simulink model "b_2x_8a_r309b"  (Simulink 6.2)
settings: Solver=ode45  StartTime=0.0  StopTime=1030.0  RelTol=1e-3
undefined symbols (not defined in the file): ant_bits, BEE2_usr, blockCountBits, blockRowBits, cmult_4bit_em
libraries: xbsIndex_r3 x3291, xps_library x101, casper_library x95
(part 2 of 22)

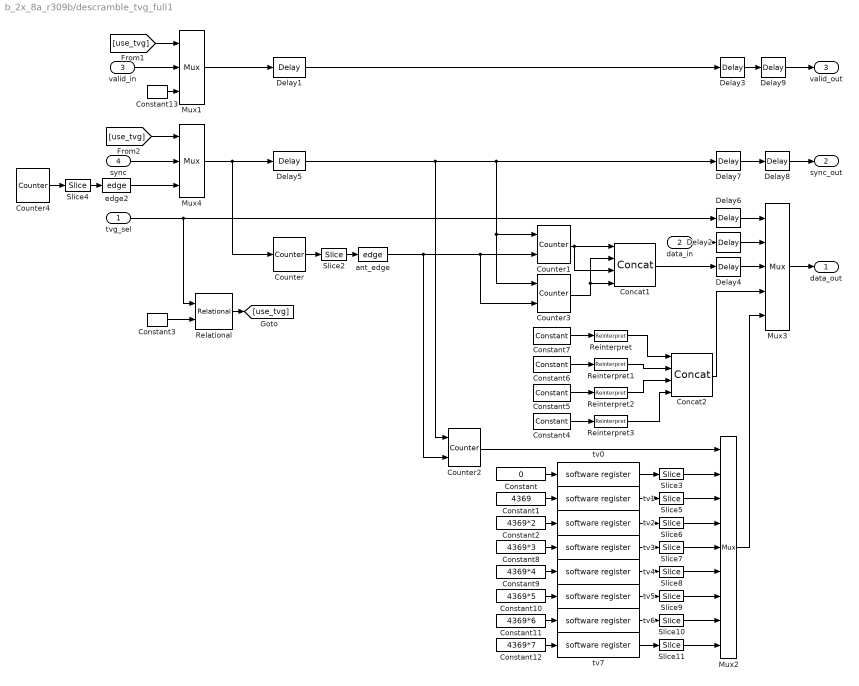
== system b_2x_8a_r309b/descramble_tvg_full1 ==
  tvg_sel : Inport  Port=1  LatchInput=off
  data_in : Inport  Port=2  LatchInput=off
  valid_in : Inport  Port=3  LatchInput=off
  sync : Inport  Port=4  LatchInput=off
  Concat1 : xbsIndex_r3/Concat  num_inputs=4  explicit_period=off  period=1  dbl_ovrd=off
  Concat2 : xbsIndex_r3/Concat  num_inputs=4  explicit_period=off  period=1  dbl_ovrd=off
  Constant : Constant  Value=0
  Constant1 : Constant  Value=4369
  Constant10 : Constant  Value=4369*5
  Constant11 : Constant  Value=4369*6
  Constant12 : Constant  Value=4369*7
  Constant13 : xbsIndex_r3/Constant  const=1  equ=P=C  arith_type=Boolean  n_bits=1  bin_pt=0  opselect=C  inp2=PCIN>>17  opr=+  inp1=P  carry=CIN  iostate=0  explicit_period=on  period=1  dbl_ovrd=off
  Constant2 : Constant  Value=4369*2
  Constant3 : xbsIndex_r3/Constant  const=0  equ=P=C  arith_type=Unsigned  n_bits=2  bin_pt=0  opselect=C  inp2=PCIN>>17  opr=+  inp1=P  carry=CIN  iostate=0  explicit_period=on  period=1  dbl_ovrd=off
  Constant4 : xbsIndex_r3/Constant  const=-0.25  equ=P=C  arith_type="Signed  (2's comp)"  n_bits=4  bin_pt=3  opselect=C  inp2=PCIN>>17  opr=+  inp1=P  carry=CIN  iostate=0  explicit_period=on  period=1  dbl_ovrd=off
  Constant5 : xbsIndex_r3/Constant  const=0.5  equ=P=C  arith_type="Signed  (2's comp)"  n_bits=4  bin_pt=3  opselect=C  inp2=PCIN>>17  opr=+  inp1=P  carry=CIN  iostate=0  explicit_period=on  period=1  dbl_ovrd=off
  Constant6 : xbsIndex_r3/Constant  const=-6/8  equ=P=C  arith_type="Signed  (2's comp)"  n_bits=4  bin_pt=3  opselect=C  inp2=PCIN>>17  opr=+  inp1=P  carry=CIN  iostate=0  explicit_period=on  period=1  dbl_ovrd=off
  Constant7 : xbsIndex_r3/Constant  const=0.1  equ=P=C  arith_type="Signed  (2's comp)"  n_bits=4  bin_pt=3  opselect=C  inp2=PCIN>>17  opr=+  inp1=P  carry=CIN  iostate=0  explicit_period=on  period=1  dbl_ovrd=off
  Constant8 : Constant  Value=4369*3
  Constant9 : Constant  Value=4369*4
  Counter : xbsIndex_r3/Counter  cnt_type=Free Running  n_bits=x_int_bits + 1  bin_pt=0  arith_type=Unsigned  start_count=0  cnt_to=Inf  cnt_by_val=1  operation=Up  explicit_period=off  period=1  load_pin=off  rst=on  en=off  dbl_ovrd=off  show_param=off  use_rpm=on  gen_core=off
      settings: xl_area=[0, 0, 0, 0, 0, 0, 0]
  Counter1 : xbsIndex_r3/Counter  cnt_type=Free Running  n_bits=4  bin_pt=0  arith_type=Unsigned  start_count=0  cnt_to=7  cnt_by_val=1  operation=Up  explicit_period=off  period=1  load_pin=off  rst=on  en=on  dbl_ovrd=off  show_param=off  use_rpm=on  gen_core=off
      settings: xl_area=[0, 0, 0, 0, 0, 0, 0]
  Counter2 : xbsIndex_r3/Counter  cnt_type=Free Running  n_bits=3  bin_pt=0  arith_type=Unsigned  start_count=0  cnt_to=7  cnt_by_val=1  operation=Up  explicit_period=off  period=1  load_pin=off  rst=on  en=on  dbl_ovrd=off  show_param=off  use_rpm=on  gen_core=off
      settings: xl_area=[0, 0, 0, 0, 0, 0, 0]
  Counter3 : xbsIndex_r3/Counter  cnt_type=Free Running  n_bits=4  bin_pt=0  arith_type=Unsigned  start_count=15  cnt_to=0  cnt_by_val=1  operation=Down  explicit_period=off  period=1  load_pin=off  rst=on  en=on  dbl_ovrd=off  show_param=off  use_rpm=on  gen_core=off
      settings: xl_area=[0, 0, 0, 0, 0, 0, 0]
  Counter4 : xbsIndex_r3/Counter  cnt_type=Free Running  n_bits=sync_period+1  bin_pt=0  arith_type=Unsigned  start_count=2^sync_period - 2  cnt_to=Inf  cnt_by_val=1  operation=Up  explicit_period=off  period=1  load_pin=off  rst=off  en=off  dbl_ovrd=off  show_param=off  use_rpm=on  gen_core=off
      settings: xl_area=[0, 0, 0, 0, 0, 0, 0]
  Delay{1,3..9} (8 alike) : xbsIndex_r3/Delay  latency=1  reg_retiming=off  explicit_period=off  period=1  en=off  accept_only_valid=off  init_zero=on  dbl_ovrd=off  show_param=off
      settings: xl_area=[0, 0, 0, 0, 0, 0, 0]
  Delay2 : xbsIndex_r3/Delay  latency=2  reg_retiming=off  explicit_period=off  period=1  en=off  accept_only_valid=off  init_zero=on  dbl_ovrd=off  show_param=off
      settings: xl_area=[0, 0, 0, 0, 0, 0, 0]
  Mux1 : xbsIndex_r3/Mux  inputs=2  precision=Full  arith_type="Signed  (2's comp)"  n_bits=8  bin_pt=2  quantization=Truncate  overflow=Wrap  latency=0  explicit_period=on  period=1  en=off  dbl_ovrd=off  show_param=off  mux_type=off  use_rpm=off  gen_core=off
      settings: xl_area=[0, 0, 0, 0, 0, 0, 0]
  Mux2 : xbsIndex_r3/Mux  inputs=8  precision=Full  arith_type="Signed  (2's comp)"  n_bits=8  bin_pt=2  quantization=Truncate  overflow=Wrap  latency=1  explicit_period=off  period=1  en=off  dbl_ovrd=off  show_param=off  mux_type=off  use_rpm=off  gen_core=off
      settings: xl_area=[0, 0, 0, 0, 0, 0, 0]
  Mux3 : xbsIndex_r3/Mux  inputs=4  precision=Full  arith_type="Signed  (2's comp)"  n_bits=8  bin_pt=2  quantization=Truncate  overflow=Wrap  latency=1  explicit_period=off  period=1  en=off  dbl_ovrd=off  show_param=off  mux_type=off  use_rpm=off  gen_core=off
      settings: xl_area=[0, 0, 0, 0, 0, 0, 0]
  Mux4 : xbsIndex_r3/Mux  inputs=2  precision=Full  arith_type="Signed  (2's comp)"  n_bits=8  bin_pt=2  quantization=Truncate  overflow=Wrap  latency=0  explicit_period=on  period=1  en=off  dbl_ovrd=off  show_param=off  mux_type=off  use_rpm=off  gen_core=off
      settings: xl_area=[0, 0, 0, 0, 0, 0, 0]
  Reinterpret{,1..3} (4 alike) : xbsIndex_r3/Reinterpret  force_arith_type=on  arith_type=Unsigned  force_bin_pt=on  bin_pt=0  force_valid=on
  Relational : xbsIndex_r3/Relational  mode=a!=b  latency=1  explicit_period=off  period=1  en=off  dbl_ovrd=off  show_param=off
      settings: xl_area=[0, 0, 0, 0, 0, 0, 0]
  Slice{3,5..11} (8 alike) : xbsIndex_r3/Slice  mode=Lower Bit Location + Width  nbits=16  bit1=0  base1=MSB of Input  bit0=0  base0=LSB of Input  boolean_output=off  explicit_period=off  period=1  dbl_ovrd=off
  Slice2 : xbsIndex_r3/Slice  mode=Lower Bit Location + Width  nbits=1  bit1=0  base1=MSB of Input  bit0=x_int_bits  base0=LSB of Input  boolean_output=on  explicit_period=off  period=1  dbl_ovrd=off
  Slice4 : xbsIndex_r3/Slice  mode=Lower Bit Location + Width  nbits=1  bit1=0  base1=MSB of Input  bit0=sync_period  base0=LSB of Input  boolean_output=on  explicit_period=off  period=1  dbl_ovrd=off
  ant_edge : casper_library/Misc/edge
  edge2 : casper_library/Misc/edge
  tv0 : xps_library/software register  Tag=xps:sw_reg  io_dir=From Processor  arith_type=Unsigned  bitwidth=32  bin_pt=0  sample_period=1  gw_name=b_2x_8a_r309b_descramble_tvg_full1_tv0_user_data_out
  tv1 : xps_library/software register  Tag=xps:sw_reg  io_dir=From Processor  arith_type=Unsigned  bitwidth=32  bin_pt=0  sample_period=1  gw_name=b_2x_8a_r309b_descramble_tvg_full1_tv1_user_data_out
  tv2 : xps_library/software register  Tag=xps:sw_reg  io_dir=From Processor  arith_type=Unsigned  bitwidth=32  bin_pt=0  sample_period=1  gw_name=b_2x_8a_r309b_descramble_tvg_full1_tv2_user_data_out
  tv3 : xps_library/software register  Tag=xps:sw_reg  io_dir=From Processor  arith_type=Unsigned  bitwidth=32  bin_pt=0  sample_period=1  gw_name=b_2x_8a_r309b_descramble_tvg_full1_tv3_user_data_out
  tv4 : xps_library/software register  Tag=xps:sw_reg  io_dir=From Processor  arith_type=Unsigned  bitwidth=32  bin_pt=0  sample_period=1  gw_name=b_2x_8a_r309b_descramble_tvg_full1_tv4_user_data_out
  tv5 : xps_library/software register  Tag=xps:sw_reg  io_dir=From Processor  arith_type=Unsigned  bitwidth=32  bin_pt=0  sample_period=1  gw_name=b_2x_8a_r309b_descramble_tvg_full1_tv5_user_data_out
  tv6 : xps_library/software register  Tag=xps:sw_reg  io_dir=From Processor  arith_type=Unsigned  bitwidth=32  bin_pt=0  sample_period=1  gw_name=b_2x_8a_r309b_descramble_tvg_full1_tv6_user_data_out
  tv7 : xps_library/software register  Tag=xps:sw_reg  io_dir=From Processor  arith_type=Unsigned  bitwidth=32  bin_pt=0  sample_period=1  gw_name=b_2x_8a_r309b_descramble_tvg_full1_tv7_user_data_out
  data_out : Outport
  sync_out : Outport  Port=2
  valid_out : Outport  Port=3
  wires:
  Counter1/1 -> Concat1/1, Concat1/3
  ant_edge/1 -> Counter2/2, Counter1/2, Counter3/2
  Counter/1 -> Slice2/1
  Slice2/1 -> ant_edge/1
  Concat1/1 -> Delay4/1
  Delay8/1 -> sync_out/1
  data_in/1 -> Delay2/1
  Delay2/1 -> Mux3/2
  Mux3/1 -> data_out/1
  Delay3/1 -> Delay9/1
  tvg_sel/1 -> Delay6/1, Relational/1
  Delay6/1 -> Mux3/1
  Constant3/1 -> Relational/2
  Concat2/1 -> Mux3/4
  Counter3/1 -> Concat1/2, Concat1/4
  Delay7/1 -> Delay8/1
  Delay5/1 -> Delay7/1, Counter1/1, Counter3/1, Counter2/1
  Delay4/1 -> Mux3/3
  Relational/1 -> [use_tvg]
  [use_tvg] -> Mux4/1
  Slice4/1 -> edge2/1
  Counter4/1 -> Slice4/1
  sync/1 -> Mux4/2
  Mux4/1 -> Delay5/1, Counter/1
  tv0/1 -> Slice3/1
  Constant/1 -> tv0/1
  Mux2/1 -> Mux3/5
  Slice3/1 -> Mux2/2
  Counter2/1 -> Mux2/1
  tv1/1 -> Slice5/1
  tv2/1 -> Slice6/1
  tv3/1 -> Slice7/1
  tv4/1 -> Slice8/1
  tv5/1 -> Slice9/1
  tv6/1 -> Slice10/1
  tv7/1 -> Slice11/1
  Slice5/1 -> Mux2/3
  Slice6/1 -> Mux2/4
  Slice7/1 -> Mux2/5
  Slice8/1 -> Mux2/6
  Slice9/1 -> Mux2/7
  Slice10/1 -> Mux2/8
  Slice11/1 -> Mux2/9
  edge2/1 -> Mux4/3
  Constant7/1 -> Reinterpret/1
  Constant6/1 -> Reinterpret1/1
  Constant5/1 -> Reinterpret2/1
  Constant4/1 -> Reinterpret3/1
  Reinterpret/1 -> Concat2/1
  Reinterpret1/1 -> Concat2/2
  Reinterpret2/1 -> Concat2/3
  Reinterpret3/1 -> Concat2/4
  Constant1/1 -> tv1/1
  Constant2/1 -> tv2/1
  Constant12/1 -> tv7/1
  Constant11/1 -> tv6/1
  Constant10/1 -> tv5/1
  Constant9/1 -> tv4/1
  Constant8/1 -> tv3/1
  Delay9/1 -> valid_out/1
  valid_in/1 -> Mux1/2
  Mux1/1 -> Delay1/1
  [use_tvg] -> Mux1/1
  Constant13/1 -> Mux1/3
  Delay1/1 -> Delay3/1

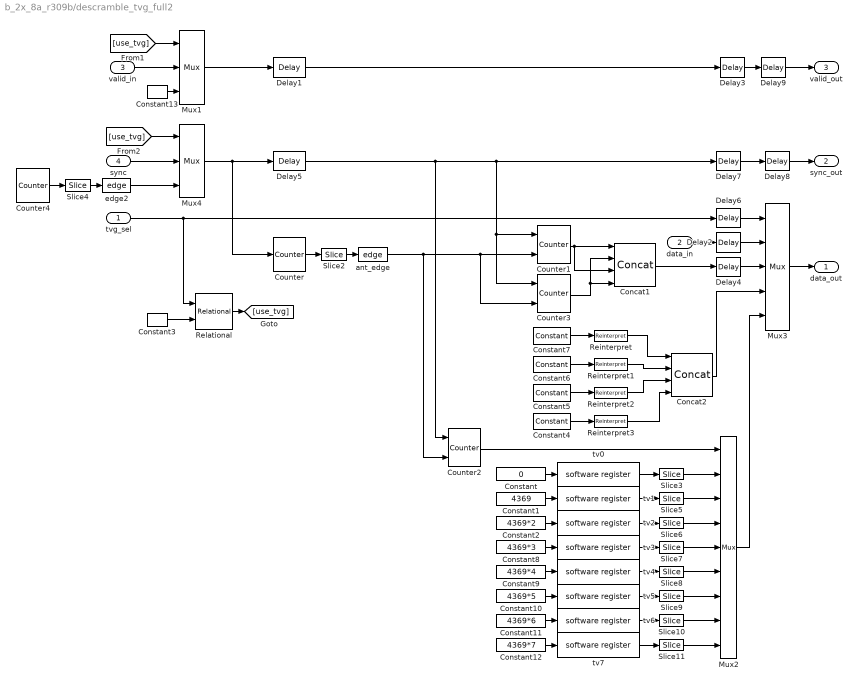
== system b_2x_8a_r309b/descramble_tvg_full2 ==
  tvg_sel : Inport  Port=1  LatchInput=off
  data_in : Inport  Port=2  LatchInput=off
  valid_in : Inport  Port=3  LatchInput=off
  sync : Inport  Port=4  LatchInput=off
  Concat1 : xbsIndex_r3/Concat  num_inputs=4  explicit_period=off  period=1  dbl_ovrd=off
  Concat2 : xbsIndex_r3/Concat  num_inputs=4  explicit_period=off  period=1  dbl_ovrd=off
  Constant : Constant  Value=0
  Constant1 : Constant  Value=4369
  Constant10 : Constant  Value=4369*5
  Constant11 : Constant  Value=4369*6
  Constant12 : Constant  Value=4369*7
  Constant13 : xbsIndex_r3/Constant  const=1  equ=P=C  arith_type=Boolean  n_bits=1  bin_pt=0  opselect=C  inp2=PCIN>>17  opr=+  inp1=P  carry=CIN  iostate=0  explicit_period=on  period=1  dbl_ovrd=off
  Constant2 : Constant  Value=4369*2
  Constant3 : xbsIndex_r3/Constant  const=0  equ=P=C  arith_type=Unsigned  n_bits=2  bin_pt=0  opselect=C  inp2=PCIN>>17  opr=+  inp1=P  carry=CIN  iostate=0  explicit_period=on  period=1  dbl_ovrd=off
  Constant4 : xbsIndex_r3/Constant  const=-0.25  equ=P=C  arith_type="Signed  (2's comp)"  n_bits=4  bin_pt=3  opselect=C  inp2=PCIN>>17  opr=+  inp1=P  carry=CIN  iostate=0  explicit_period=on  period=1  dbl_ovrd=off
  Constant5 : xbsIndex_r3/Constant  const=0.5  equ=P=C  arith_type="Signed  (2's comp)"  n_bits=4  bin_pt=3  opselect=C  inp2=PCIN>>17  opr=+  inp1=P  carry=CIN  iostate=0  explicit_period=on  period=1  dbl_ovrd=off
  Constant6 : xbsIndex_r3/Constant  const=-6/8  equ=P=C  arith_type="Signed  (2's comp)"  n_bits=4  bin_pt=3  opselect=C  inp2=PCIN>>17  opr=+  inp1=P  carry=CIN  iostate=0  explicit_period=on  period=1  dbl_ovrd=off
  Constant7 : xbsIndex_r3/Constant  const=0.1  equ=P=C  arith_type="Signed  (2's comp)"  n_bits=4  bin_pt=3  opselect=C  inp2=PCIN>>17  opr=+  inp1=P  carry=CIN  iostate=0  explicit_period=on  period=1  dbl_ovrd=off
  Constant8 : Constant  Value=4369*3
  Constant9 : Constant  Value=4369*4
  Counter : xbsIndex_r3/Counter  cnt_type=Free Running  n_bits=x_int_bits + 1  bin_pt=0  arith_type=Unsigned  start_count=0  cnt_to=Inf  cnt_by_val=1  operation=Up  explicit_period=off  period=1  load_pin=off  rst=on  en=off  dbl_ovrd=off  show_param=off  use_rpm=on  gen_core=off
      settings: xl_area=[0, 0, 0, 0, 0, 0, 0]
  Counter1 : xbsIndex_r3/Counter  cnt_type=Free Running  n_bits=4  bin_pt=0  arith_type=Unsigned  start_count=0  cnt_to=7  cnt_by_val=1  operation=Up  explicit_period=off  period=1  load_pin=off  rst=on  en=on  dbl_ovrd=off  show_param=off  use_rpm=on  gen_core=off
      settings: xl_area=[0, 0, 0, 0, 0, 0, 0]
  Counter2 : xbsIndex_r3/Counter  cnt_type=Free Running  n_bits=3  bin_pt=0  arith_type=Unsigned  start_count=0  cnt_to=7  cnt_by_val=1  operation=Up  explicit_period=off  period=1  load_pin=off  rst=on  en=on  dbl_ovrd=off  show_param=off  use_rpm=on  gen_core=off
      settings: xl_area=[0, 0, 0, 0, 0, 0, 0]
  Counter3 : xbsIndex_r3/Counter  cnt_type=Free Running  n_bits=4  bin_pt=0  arith_type=Unsigned  start_count=15  cnt_to=0  cnt_by_val=1  operation=Down  explicit_period=off  period=1  load_pin=off  rst=on  en=on  dbl_ovrd=off  show_param=off  use_rpm=on  gen_core=off
      settings: xl_area=[0, 0, 0, 0, 0, 0, 0]
  Counter4 : xbsIndex_r3/Counter  cnt_type=Free Running  n_bits=sync_period+1  bin_pt=0  arith_type=Unsigned  start_count=2^sync_period - 2  cnt_to=Inf  cnt_by_val=1  operation=Up  explicit_period=off  period=1  load_pin=off  rst=off  en=off  dbl_ovrd=off  show_param=off  use_rpm=on  gen_core=off
      settings: xl_area=[0, 0, 0, 0, 0, 0, 0]
  Delay{1,3..9} (8 alike) : xbsIndex_r3/Delay  latency=1  reg_retiming=off  explicit_period=off  period=1  en=off  accept_only_valid=off  init_zero=on  dbl_ovrd=off  show_param=off
      settings: xl_area=[0, 0, 0, 0, 0, 0, 0]
  Delay2 : xbsIndex_r3/Delay  latency=2  reg_retiming=off  explicit_period=off  period=1  en=off  accept_only_valid=off  init_zero=on  dbl_ovrd=off  show_param=off
      settings: xl_area=[0, 0, 0, 0, 0, 0, 0]
  Mux1 : xbsIndex_r3/Mux  inputs=2  precision=Full  arith_type="Signed  (2's comp)"  n_bits=8  bin_pt=2  quantization=Truncate  overflow=Wrap  latency=0  explicit_period=on  period=1  en=off  dbl_ovrd=off  show_param=off  mux_type=off  use_rpm=off  gen_core=off
      settings: xl_area=[0, 0, 0, 0, 0, 0, 0]
  Mux2 : xbsIndex_r3/Mux  inputs=8  precision=Full  arith_type="Signed  (2's comp)"  n_bits=8  bin_pt=2  quantization=Truncate  overflow=Wrap  latency=1  explicit_period=off  period=1  en=off  dbl_ovrd=off  show_param=off  mux_type=off  use_rpm=off  gen_core=off
      settings: xl_area=[0, 0, 0, 0, 0, 0, 0]
  Mux3 : xbsIndex_r3/Mux  inputs=4  precision=Full  arith_type="Signed  (2's comp)"  n_bits=8  bin_pt=2  quantization=Truncate  overflow=Wrap  latency=1  explicit_period=off  period=1  en=off  dbl_ovrd=off  show_param=off  mux_type=off  use_rpm=off  gen_core=off
      settings: xl_area=[0, 0, 0, 0, 0, 0, 0]
  Mux4 : xbsIndex_r3/Mux  inputs=2  precision=Full  arith_type="Signed  (2's comp)"  n_bits=8  bin_pt=2  quantization=Truncate  overflow=Wrap  latency=0  explicit_period=on  period=1  en=off  dbl_ovrd=off  show_param=off  mux_type=off  use_rpm=off  gen_core=off
      settings: xl_area=[0, 0, 0, 0, 0, 0, 0]
  Reinterpret{,1..3} (4 alike) : xbsIndex_r3/Reinterpret  force_arith_type=on  arith_type=Unsigned  force_bin_pt=on  bin_pt=0  force_valid=on
  Relational : xbsIndex_r3/Relational  mode=a!=b  latency=1  explicit_period=off  period=1  en=off  dbl_ovrd=off  show_param=off
      settings: xl_area=[0, 0, 0, 0, 0, 0, 0]
  Slice{3,5..11} (8 alike) : xbsIndex_r3/Slice  mode=Lower Bit Location + Width  nbits=16  bit1=0  base1=MSB of Input  bit0=0  base0=LSB of Input  boolean_output=off  explicit_period=off  period=1  dbl_ovrd=off
  Slice2 : xbsIndex_r3/Slice  mode=Lower Bit Location + Width  nbits=1  bit1=0  base1=MSB of Input  bit0=x_int_bits  base0=LSB of Input  boolean_output=on  explicit_period=off  period=1  dbl_ovrd=off
  Slice4 : xbsIndex_r3/Slice  mode=Lower Bit Location + Width  nbits=1  bit1=0  base1=MSB of Input  bit0=sync_period  base0=LSB of Input  boolean_output=on  explicit_period=off  period=1  dbl_ovrd=off
  ant_edge : casper_library/Misc/edge
  edge2 : casper_library/Misc/edge
  tv0 : xps_library/software register  Tag=xps:sw_reg  io_dir=From Processor  arith_type=Unsigned  bitwidth=32  bin_pt=0  sample_period=1  gw_name=b_2x_8a_r309b_descramble_tvg_full2_tv0_user_data_out
  tv1 : xps_library/software register  Tag=xps:sw_reg  io_dir=From Processor  arith_type=Unsigned  bitwidth=32  bin_pt=0  sample_period=1  gw_name=b_2x_8a_r309b_descramble_tvg_full2_tv1_user_data_out
  tv2 : xps_library/software register  Tag=xps:sw_reg  io_dir=From Processor  arith_type=Unsigned  bitwidth=32  bin_pt=0  sample_period=1  gw_name=b_2x_8a_r309b_descramble_tvg_full2_tv2_user_data_out
  tv3 : xps_library/software register  Tag=xps:sw_reg  io_dir=From Processor  arith_type=Unsigned  bitwidth=32  bin_pt=0  sample_period=1  gw_name=b_2x_8a_r309b_descramble_tvg_full2_tv3_user_data_out
  tv4 : xps_library/software register  Tag=xps:sw_reg  io_dir=From Processor  arith_type=Unsigned  bitwidth=32  bin_pt=0  sample_period=1  gw_name=b_2x_8a_r309b_descramble_tvg_full2_tv4_user_data_out
  tv5 : xps_library/software register  Tag=xps:sw_reg  io_dir=From Processor  arith_type=Unsigned  bitwidth=32  bin_pt=0  sample_period=1  gw_name=b_2x_8a_r309b_descramble_tvg_full2_tv5_user_data_out
  tv6 : xps_library/software register  Tag=xps:sw_reg  io_dir=From Processor  arith_type=Unsigned  bitwidth=32  bin_pt=0  sample_period=1  gw_name=b_2x_8a_r309b_descramble_tvg_full2_tv6_user_data_out
  tv7 : xps_library/software register  Tag=xps:sw_reg  io_dir=From Processor  arith_type=Unsigned  bitwidth=32  bin_pt=0  sample_period=1  gw_name=b_2x_8a_r309b_descramble_tvg_full2_tv7_user_data_out
  data_out : Outport
  sync_out : Outport  Port=2
  valid_out : Outport  Port=3
  wires:
  Counter1/1 -> Concat1/1, Concat1/3
  ant_edge/1 -> Counter2/2, Counter1/2, Counter3/2
  Counter/1 -> Slice2/1
  Slice2/1 -> ant_edge/1
  Concat1/1 -> Delay4/1
  Delay8/1 -> sync_out/1
  data_in/1 -> Delay2/1
  Delay2/1 -> Mux3/2
  Mux3/1 -> data_out/1
  Delay3/1 -> Delay9/1
  tvg_sel/1 -> Delay6/1, Relational/1
  Delay6/1 -> Mux3/1
  Constant3/1 -> Relational/2
  Concat2/1 -> Mux3/4
  Counter3/1 -> Concat1/2, Concat1/4
  Delay7/1 -> Delay8/1
  Delay5/1 -> Delay7/1, Counter1/1, Counter3/1, Counter2/1
  Delay4/1 -> Mux3/3
  Relational/1 -> [use_tvg]
  [use_tvg] -> Mux4/1
  Slice4/1 -> edge2/1
  Counter4/1 -> Slice4/1
  sync/1 -> Mux4/2
  Mux4/1 -> Delay5/1, Counter/1
  tv0/1 -> Slice3/1
  Constant/1 -> tv0/1
  Mux2/1 -> Mux3/5
  Slice3/1 -> Mux2/2
  Counter2/1 -> Mux2/1
  tv1/1 -> Slice5/1
  tv2/1 -> Slice6/1
  tv3/1 -> Slice7/1
  tv4/1 -> Slice8/1
  tv5/1 -> Slice9/1
  tv6/1 -> Slice10/1
  tv7/1 -> Slice11/1
  Slice5/1 -> Mux2/3
  Slice6/1 -> Mux2/4
  Slice7/1 -> Mux2/5
  Slice8/1 -> Mux2/6
  Slice9/1 -> Mux2/7
  Slice10/1 -> Mux2/8
  Slice11/1 -> Mux2/9
  edge2/1 -> Mux4/3
  Constant7/1 -> Reinterpret/1
  Constant6/1 -> Reinterpret1/1
  Constant5/1 -> Reinterpret2/1
  Constant4/1 -> Reinterpret3/1
  Reinterpret/1 -> Concat2/1
  Reinterpret1/1 -> Concat2/2
  Reinterpret2/1 -> Concat2/3
  Reinterpret3/1 -> Concat2/4
  Constant1/1 -> tv1/1
  Constant2/1 -> tv2/1
  Constant12/1 -> tv7/1
  Constant11/1 -> tv6/1
  Constant10/1 -> tv5/1
  Constant9/1 -> tv4/1
  Constant8/1 -> tv3/1
  Delay9/1 -> valid_out/1
  valid_in/1 -> Mux1/2
  Mux1/1 -> Delay1/1
  [use_tvg] -> Mux1/1
  Constant13/1 -> Mux1/3
  Delay1/1 -> Delay3/1

== system b_2x_8a_r309b/descramble_window1 ==
  note: BRAM depth is
      | X int length * # antennas * # windows
  din : Inport  Port=1  LatchInput=off
  we : Inport  Port=2  LatchInput=off
  eof : Inport  Port=3  LatchInput=off
  mcnt : Inport  Port=4  LatchInput=off
  ant : Inport  Port=5  LatchInput=off
  flag : Inport  Port=6  LatchInput=off
  Constant : xbsIndex_r3/Constant  const=0  equ=P=C  arith_type=Unsigned  n_bits=18  bin_pt=0  opselect=C  inp2=PCIN>>17  opr=+  inp1=P  carry=CIN  iostate=0  explicit_period=on  period=1  dbl_ovrd=off
  Delay1 : xbsIndex_r3/Delay  latency=2  reg_retiming=off  explicit_period=off  period=1  en=off  accept_only_valid=off  init_zero=on  dbl_ovrd=off  show_param=off
      settings: xl_area=[0, 0, 0, 0, 0, 0, 0]
  Delay2 : xbsIndex_r3/Delay  latency=4  reg_retiming=off  explicit_period=off  period=1  en=off  accept_only_valid=off  init_zero=on  dbl_ovrd=off  show_param=off
      settings: xl_area=[0, 0, 0, 0, 0, 0, 0]
  Delay3 : xbsIndex_r3/Delay  latency=2  reg_retiming=off  explicit_period=off  period=1  en=off  accept_only_valid=off  init_zero=on  dbl_ovrd=off  show_param=off
      settings: xl_area=[0, 0, 0, 0, 0, 0, 0]
  Delay4 : xbsIndex_r3/Delay  latency=4  reg_retiming=off  explicit_period=off  period=1  en=off  accept_only_valid=off  init_zero=on  dbl_ovrd=off  show_param=off
      settings: xl_area=[0, 0, 0, 0, 0, 0, 0]
  Dual Port RAM : xbsIndex_r3/Dual Port RAM  depth=2^x_int_bits * 2^ant_bits * 2^window_bits  initVector=0  write_mode_A=Read Before Write  write_mode_B=Read Before Write  latency=2  mem_collision=off  init_zero=on  explicit_period=off  period=1  dbl_ovrd=off  rst_a=off  init_a=0  rst_b=off  init_b=0  show_param=off  distributed_mem=off  use_rpm=off  gen_core=off
      settings: xl_area=[0, 0, 0, 0, 0, 0, 0]
  Terminator : Terminator
  deflagger : Subsystem
  flagger : Subsystem
  window_addr_gen : Subsystem
  dout : Outport
  valid : Outport  Port=2
  flag_out : Outport  Port=3
  rcvd : Outport  Port=4
  sync_out : Outport  Port=5
  wires:
  Dual Port RAM/2 -> Terminator/1
  Dual Port RAM/1 -> deflagger/1(din)
  window_addr_gen/4(we) -> Dual Port RAM/6
  window_addr_gen/3(wr_addr) -> Dual Port RAM/4
  window_addr_gen/2(re) -> Dual Port RAM/3, Delay1/1
  window_addr_gen/1(rd_addr) -> Dual Port RAM/1
  flagger/1(dout) -> Dual Port RAM/5
  Constant/1 -> Dual Port RAM/2
  deflagger/3(rcvd) -> rcvd/1
  deflagger/2(flag) -> flag_out/1
  deflagger/1(dout) -> dout/1
  Delay1/1 -> valid/1
  we/1 -> window_addr_gen/4(valid)
  eof/1 -> window_addr_gen/3(eof)
  ant/1 -> window_addr_gen/2(ant)
  mcnt/1 -> window_addr_gen/1(mcnt)
  Delay3/1 -> sync_out/1
  window_addr_gen/5(sync_out) -> Delay3/1
  flag/1 -> Delay4/1
  Delay4/1 -> flagger/1(flag)
  din/1 -> Delay2/1
  Delay2/1 -> flagger/2(din)

== system b_2x_8a_r309b/descramble_window2 ==
  note: BRAM depth is
      | X int length * # antennas * # windows
  din : Inport  Port=1  LatchInput=off
  we : Inport  Port=2  LatchInput=off
  eof : Inport  Port=3  LatchInput=off
  mcnt : Inport  Port=4  LatchInput=off
  ant : Inport  Port=5  LatchInput=off
  flag : Inport  Port=6  LatchInput=off
  Constant : xbsIndex_r3/Constant  const=0  equ=P=C  arith_type=Unsigned  n_bits=18  bin_pt=0  opselect=C  inp2=PCIN>>17  opr=+  inp1=P  carry=CIN  iostate=0  explicit_period=on  period=1  dbl_ovrd=off
  Delay1 : xbsIndex_r3/Delay  latency=2  reg_retiming=off  explicit_period=off  period=1  en=off  accept_only_valid=off  init_zero=on  dbl_ovrd=off  show_param=off
      settings: xl_area=[0, 0, 0, 0, 0, 0, 0]
  Delay2 : xbsIndex_r3/Delay  latency=4  reg_retiming=off  explicit_period=off  period=1  en=off  accept_only_valid=off  init_zero=on  dbl_ovrd=off  show_param=off
      settings: xl_area=[0, 0, 0, 0, 0, 0, 0]
  Delay3 : xbsIndex_r3/Delay  latency=2  reg_retiming=off  explicit_period=off  period=1  en=off  accept_only_valid=off  init_zero=on  dbl_ovrd=off  show_param=off
      settings: xl_area=[0, 0, 0, 0, 0, 0, 0]
  Delay4 : xbsIndex_r3/Delay  latency=4  reg_retiming=off  explicit_period=off  period=1  en=off  accept_only_valid=off  init_zero=on  dbl_ovrd=off  show_param=off
      settings: xl_area=[0, 0, 0, 0, 0, 0, 0]
  Dual Port RAM : xbsIndex_r3/Dual Port RAM  depth=2^x_int_bits * 2^ant_bits * 2^window_bits  initVector=0  write_mode_A=Read Before Write  write_mode_B=Read Before Write  latency=2  mem_collision=off  init_zero=on  explicit_period=off  period=1  dbl_ovrd=off  rst_a=off  init_a=0  rst_b=off  init_b=0  show_param=off  distributed_mem=off  use_rpm=off  gen_core=off
      settings: xl_area=[0, 0, 0, 0, 0, 0, 0]
  Terminator : Terminator
  deflagger : Subsystem
  flagger : Subsystem
  window_addr_gen : Subsystem
  dout : Outport
  valid : Outport  Port=2
  flag_out : Outport  Port=3
  rcvd : Outport  Port=4
  sync_out : Outport  Port=5
  wires:
  Delay2/1 -> flagger/2(din)
  din/1 -> Delay2/1
  Delay4/1 -> flagger/1(flag)
  flag/1 -> Delay4/1
  window_addr_gen/5(sync_out) -> Delay3/1
  Delay3/1 -> sync_out/1
  mcnt/1 -> window_addr_gen/1(mcnt)
  ant/1 -> window_addr_gen/2(ant)
  eof/1 -> window_addr_gen/3(eof)
  we/1 -> window_addr_gen/4(valid)
  Delay1/1 -> valid/1
  deflagger/1(dout) -> dout/1
  deflagger/2(flag) -> flag_out/1
  deflagger/3(rcvd) -> rcvd/1
  Constant/1 -> Dual Port RAM/2
  flagger/1(dout) -> Dual Port RAM/5
  window_addr_gen/1(rd_addr) -> Dual Port RAM/1
  window_addr_gen/2(re) -> Delay1/1, Dual Port RAM/3
  window_addr_gen/3(wr_addr) -> Dual Port RAM/4
  window_addr_gen/4(we) -> Dual Port RAM/6
  Dual Port RAM/1 -> deflagger/1(din)
  Dual Port RAM/2 -> Terminator/1

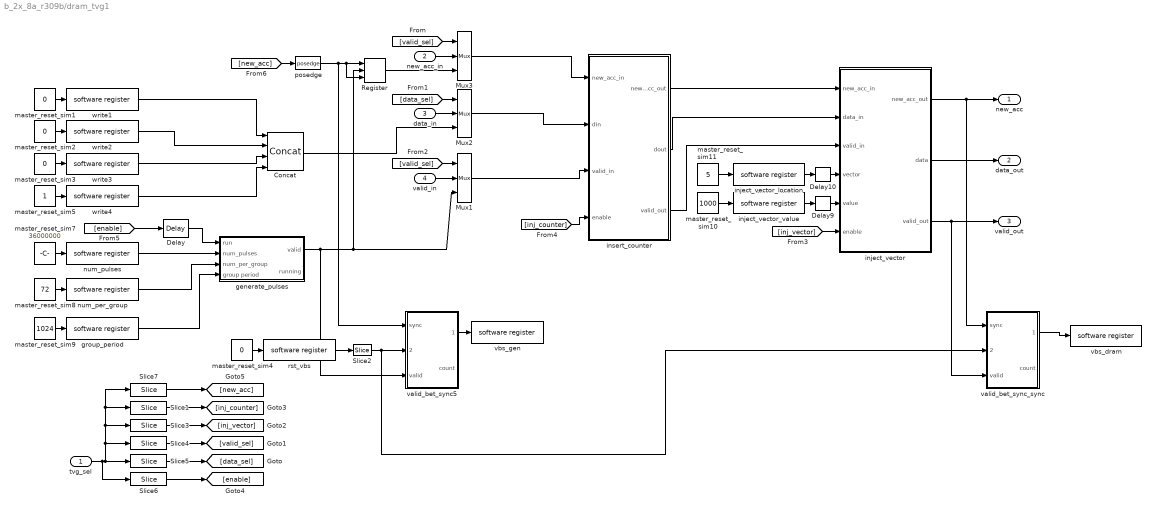
== system b_2x_8a_r309b/dram_tvg1 ==
  tvg_sel : Inport  Port=1  LatchInput=off
  new_acc_in : Inport  Port=2  LatchInput=off
  data_in : Inport  Port=3  LatchInput=off
  valid_in : Inport  Port=4  LatchInput=off
  Concat : xbsIndex_r3/Concat  num_inputs=4  explicit_period=on  period=1  dbl_ovrd=off
  Delay : xbsIndex_r3/Delay  latency=1  reg_retiming=on  explicit_period=off  period=1  en=off  accept_only_valid=off  init_zero=on  dbl_ovrd=off  show_param=off
      settings: xl_area=[0, 0, 0, 0, 0, 0, 0]
  Delay10 : xbsIndex_r3/Delay  latency=5  reg_retiming=off  explicit_period=off  period=1  en=off  accept_only_valid=off  init_zero=on  dbl_ovrd=off  show_param=off
      settings: xl_area=[0, 0, 0, 0, 0, 0, 0]
  Delay9 : xbsIndex_r3/Delay  latency=5  reg_retiming=off  explicit_period=off  period=1  en=off  accept_only_valid=off  init_zero=on  dbl_ovrd=off  show_param=off
      settings: xl_area=[0, 0, 0, 0, 0, 0, 0]
  Mux1 : xbsIndex_r3/Mux  inputs=2  precision=Full  arith_type="Signed  (2's comp)"  n_bits=8  bin_pt=2  quantization=Truncate  overflow=Wrap  latency=0  explicit_period=off  period=1  en=off  dbl_ovrd=off  show_param=off  mux_type=off  use_rpm=off  gen_core=off
      settings: xl_area=[0, 0, 0, 0, 0, 0, 0]
  Mux2 : xbsIndex_r3/Mux  inputs=2  precision=Full  arith_type="Signed  (2's comp)"  n_bits=8  bin_pt=2  quantization=Truncate  overflow=Wrap  latency=0  explicit_period=off  period=1  en=off  dbl_ovrd=off  show_param=off  mux_type=off  use_rpm=off  gen_core=off
      settings: xl_area=[0, 0, 0, 0, 0, 0, 0]
  Mux3 : xbsIndex_r3/Mux  inputs=2  precision=Full  arith_type="Signed  (2's comp)"  n_bits=8  bin_pt=2  quantization=Truncate  overflow=Wrap  latency=0  explicit_period=off  period=1  en=off  dbl_ovrd=off  show_param=off  mux_type=off  use_rpm=off  gen_core=off
      settings: xl_area=[0, 0, 0, 0, 0, 0, 0]
  Register : xbsIndex_r3/Register  init=0  reg_only_valid=off  explicit_period=off  period=1  rst=on  en=on  out_en=off  dbl_ovrd=off  show_param=off
      settings: xl_area=[0, 0, 0, 0, 0, 0, 0]
  Slice1 : xbsIndex_r3/Slice  mode=Lower Bit Location + Width  nbits=1  bit1=0  base1=MSB of Input  bit0=4  base0=LSB of Input  boolean_output=on  explicit_period=off  period=1  dbl_ovrd=off
  Slice2 : xbsIndex_r3/Slice  mode=Lower Bit Location + Width  nbits=1  bit1=0  base1=MSB of Input  bit0=0  base0=LSB of Input  boolean_output=on  explicit_period=off  period=1  dbl_ovrd=off
  Slice3 : xbsIndex_r3/Slice  mode=Lower Bit Location + Width  nbits=1  bit1=0  base1=MSB of Input  bit0=3  base0=LSB of Input  boolean_output=on  explicit_period=off  period=1  dbl_ovrd=off
  Slice4 : xbsIndex_r3/Slice  mode=Lower Bit Location + Width  nbits=1  bit1=0  base1=MSB of Input  bit0=2  base0=LSB of Input  boolean_output=on  explicit_period=off  period=1  dbl_ovrd=off
  Slice5 : xbsIndex_r3/Slice  mode=Lower Bit Location + Width  nbits=1  bit1=0  base1=MSB of Input  bit0=1  base0=LSB of Input  boolean_output=on  explicit_period=off  period=1  dbl_ovrd=off
  Slice6 : xbsIndex_r3/Slice  mode=Lower Bit Location + Width  nbits=1  bit1=0  base1=MSB of Input  bit0=0  base0=LSB of Input  boolean_output=on  explicit_period=off  period=1  dbl_ovrd=off
  Slice7 : xbsIndex_r3/Slice  mode=Lower Bit Location + Width  nbits=1  bit1=0  base1=MSB of Input  bit0=5  base0=LSB of Input  boolean_output=on  explicit_period=off  period=1  dbl_ovrd=off
  generate_pulses : Subsystem
  group_period : xps_library/software register  Tag=xps:sw_reg  io_dir=From Processor  arith_type=Unsigned  bitwidth=32  bin_pt=0  sample_period=1  gw_name=b_2x_8a_r309b_dram_tvg1_group_period_user_data_out
  inject_vector : Subsystem  mask{num_vectors=len}
      mask prompts: num_vectors "number of vectors"
      mask init:
      | fmtstr = sprintf('Vector Length: %d', num_vectors);
      | set_param(gcb, 'AttributesFormatString', fmtstr);
      settings: AttributesFormatString=Vector Length: 18432
  inject_vector_location : xps_library/software register  Tag=xps:sw_reg  io_dir=From Processor  arith_type=Unsigned  bitwidth=32  bin_pt=0  sample_period=1  gw_name=b_2x_8a_r309b_dram_tvg1_inject_vector_location_user_data_out
  inject_vector_value : xps_library/software register  Tag=xps:sw_reg  io_dir=From Processor  arith_type=Unsigned  bitwidth=32  bin_pt=0  sample_period=1  gw_name=b_2x_8a_r309b_dram_tvg1_inject_vector_value_user_data_out
  insert_counter : Subsystem  mask{vec_len=len}
      mask prompts: vec_len "Vector Length?"
      mask init:
      | fmtstr = sprintf('Vector Length: %d', vec_len);
      | set_param(gcb, 'AttributesFormatString', fmtstr);
      settings: AttributesFormatString=Vector Length: 18432
  master_reset_sim{1..4} (4 alike) : Constant  Value=0
  master_reset_sim10 : Constant  Value=1000
  master_reset_sim11 : Constant  Value=5
  master_reset_sim5 : Constant
  master_reset_sim7 : Constant  Value=36000000
  master_reset_sim8 : Constant  Value=72
  master_reset_sim9 : Constant  Value=1024
  num_per_group : xps_library/software register  Tag=xps:sw_reg  io_dir=From Processor  arith_type=Unsigned  bitwidth=32  bin_pt=0  sample_period=1  gw_name=b_2x_8a_r309b_dram_tvg1_num_per_group_user_data_out
  num_pulses : xps_library/software register  Tag=xps:sw_reg  io_dir=From Processor  arith_type=Unsigned  bitwidth=32  bin_pt=0  sample_period=1  gw_name=b_2x_8a_r309b_dram_tvg1_num_pulses_user_data_out
  posedge : casper_library/Misc/posedge  Tag=Rising Edge Detector
  rst_vbs : xps_library/software register  Tag=xps:sw_reg  io_dir=From Processor  arith_type=Unsigned  bitwidth=32  bin_pt=0  sample_period=1  gw_name=b_2x_8a_r309b_dram_tvg1_rst_vbs_user_data_out
  valid_bet_sync5 : Subsystem
  valid_bet_sync_sync : Subsystem
  vbs_dram : xps_library/software register  Tag=xps:sw_reg  io_dir=To Processor  arith_type=Unsigned  bitwidth=32  bin_pt=0  sample_period=1  gw_name=b_2x_8a_r309b_dram_tvg1_vbs_dram_user_data_in
  vbs_gen : xps_library/software register  Tag=xps:sw_reg  io_dir=To Processor  arith_type=Unsigned  bitwidth=32  bin_pt=0  sample_period=1  gw_name=b_2x_8a_r309b_dram_tvg1_vbs_gen_user_data_in
  write1 : xps_library/software register  Tag=xps:sw_reg  io_dir=From Processor  arith_type=Unsigned  bitwidth=32  bin_pt=0  sample_period=1  gw_name=b_2x_8a_r309b_dram_tvg1_write1_user_data_out
  write2 : xps_library/software register  Tag=xps:sw_reg  io_dir=From Processor  arith_type=Unsigned  bitwidth=32  bin_pt=0  sample_period=1  gw_name=b_2x_8a_r309b_dram_tvg1_write2_user_data_out
  write3 : xps_library/software register  Tag=xps:sw_reg  io_dir=From Processor  arith_type=Unsigned  bitwidth=32  bin_pt=0  sample_period=1  gw_name=b_2x_8a_r309b_dram_tvg1_write3_user_data_out
  write4 : xps_library/software register  Tag=xps:sw_reg  io_dir=From Processor  arith_type=Unsigned  bitwidth=32  bin_pt=0  sample_period=1  gw_name=b_2x_8a_r309b_dram_tvg1_write4_user_data_out
  new_acc : Outport
  data_out : Outport  Port=2
  valid_out : Outport  Port=3
  wires:
  write1/1 -> Concat/1
  master_reset_sim1/1 -> write1/1
  write2/1 -> Concat/2
  master_reset_sim2/1 -> write2/1
  write3/1 -> Concat/3
  master_reset_sim3/1 -> write3/1
  write4/1 -> Concat/4
  master_reset_sim5/1 -> write4/1
  [new_acc] -> posedge/1
  num_pulses/1 -> generate_pulses/2(num_pulses)
  master_reset_sim7/1 -> num_pulses/1
  num_per_group/1 -> generate_pulses/3(num_per_group)
  master_reset_sim8/1 -> num_per_group/1
  group_period/1 -> generate_pulses/4(group period)
  master_reset_sim9/1 -> group_period/1
  Mux1/1 -> insert_counter/3(valid_in)
  valid_in/1 -> Mux1/2
  inject_vector/1(new_acc_out) -> new_acc/1, valid_bet_sync_sync/1(sync)
  inject_vector/2(data) -> data_out/1
  inject_vector/3(valid_out) -> valid_out/1, valid_bet_sync_sync/3(valid)
  insert_counter/1(new_acc_out) -> inject_vector/1(new_acc_in)
  Mux2/1 -> insert_counter/2(din)
  data_in/1 -> Mux2/2
  new_acc_in/1 -> Mux3/2
  Mux3/1 -> insert_counter/1(new_acc_in)
  Slice5/1 -> [data_sel]
  tvg_sel/1 -> Slice5/1, Slice3/1, Slice1/1, Slice7/1, Slice4/1, Slice6/1
  Slice4/1 -> [valid_sel]
  [valid_sel] -> Mux3/1
  [data_sel] -> Mux2/1
  [valid_sel] -> Mux1/1
  Slice3/1 -> [inj_vector]
  Slice1/1 -> [inj_counter]
  [enable] -> Delay/1
  insert_counter/2(dout) -> inject_vector/2(data_in)
  insert_counter/3(valid_out) -> inject_vector/3(valid_in)
  Concat/1 -> Mux2/3
  generate_pulses/1(valid) -> Register/2, Mux1/3, valid_bet_sync5/3(valid)
  Register/1 -> Mux3/3
  posedge/1 -> Register/1, Register/3, valid_bet_sync5/1(sync)
  [inj_vector] -> inject_vector/6(enable)
  Delay10/1 -> inject_vector/4(vector)
  master_reset_sim11/1 -> inject_vector_location/1
  inject_vector_location/1 -> Delay10/1
  Delay9/1 -> inject_vector/5(value)
  master_reset_sim10/1 -> inject_vector_value/1
  inject_vector_value/1 -> Delay9/1
  [inj_counter] -> insert_counter/4(enable)
  Slice6/1 -> [enable]
  Slice7/1 -> [new_acc]
  valid_bet_sync5/1(max_count) -> vbs_gen/1
  master_reset_sim4/1 -> rst_vbs/1
  Slice2/1 -> valid_bet_sync5/2(rst_max), valid_bet_sync_sync/2(rst_max)
  rst_vbs/1 -> Slice2/1
  valid_bet_sync_sync/1(max_count) -> vbs_dram/1
  Delay/1 -> generate_pulses/1(run)

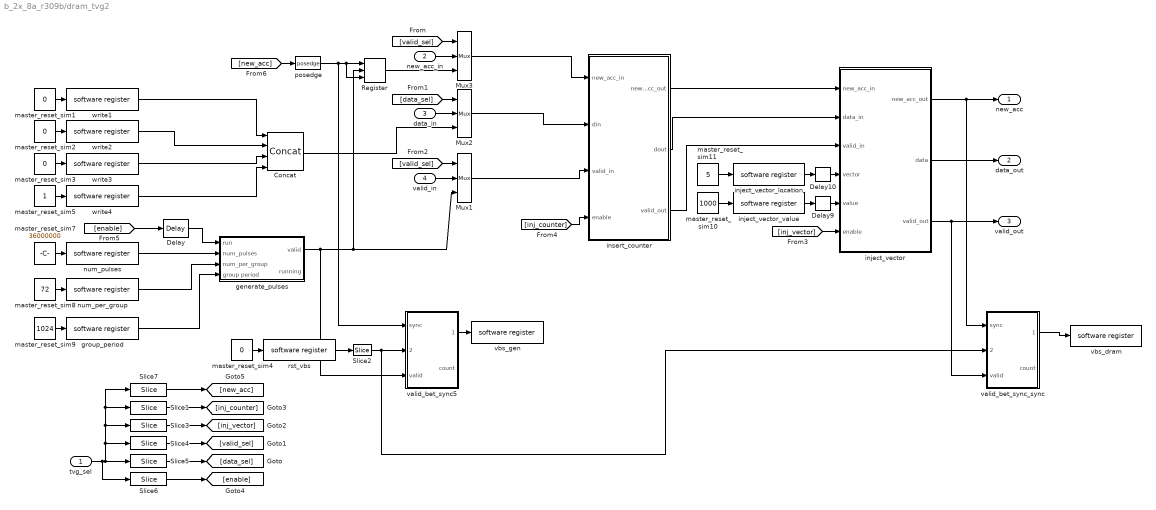
== system b_2x_8a_r309b/dram_tvg2 ==
  tvg_sel : Inport  Port=1  LatchInput=off
  new_acc_in : Inport  Port=2  LatchInput=off
  data_in : Inport  Port=3  LatchInput=off
  valid_in : Inport  Port=4  LatchInput=off
  Concat : xbsIndex_r3/Concat  num_inputs=4  explicit_period=on  period=1  dbl_ovrd=off
  Delay : xbsIndex_r3/Delay  latency=1  reg_retiming=on  explicit_period=off  period=1  en=off  accept_only_valid=off  init_zero=on  dbl_ovrd=off  show_param=off
      settings: xl_area=[0, 0, 0, 0, 0, 0, 0]
  Delay10 : xbsIndex_r3/Delay  latency=5  reg_retiming=off  explicit_period=off  period=1  en=off  accept_only_valid=off  init_zero=on  dbl_ovrd=off  show_param=off
      settings: xl_area=[0, 0, 0, 0, 0, 0, 0]
  Delay9 : xbsIndex_r3/Delay  latency=5  reg_retiming=off  explicit_period=off  period=1  en=off  accept_only_valid=off  init_zero=on  dbl_ovrd=off  show_param=off
      settings: xl_area=[0, 0, 0, 0, 0, 0, 0]
  Mux1 : xbsIndex_r3/Mux  inputs=2  precision=Full  arith_type="Signed  (2's comp)"  n_bits=8  bin_pt=2  quantization=Truncate  overflow=Wrap  latency=0  explicit_period=off  period=1  en=off  dbl_ovrd=off  show_param=off  mux_type=off  use_rpm=off  gen_core=off
      settings: xl_area=[0, 0, 0, 0, 0, 0, 0]
  Mux2 : xbsIndex_r3/Mux  inputs=2  precision=Full  arith_type="Signed  (2's comp)"  n_bits=8  bin_pt=2  quantization=Truncate  overflow=Wrap  latency=0  explicit_period=off  period=1  en=off  dbl_ovrd=off  show_param=off  mux_type=off  use_rpm=off  gen_core=off
      settings: xl_area=[0, 0, 0, 0, 0, 0, 0]
  Mux3 : xbsIndex_r3/Mux  inputs=2  precision=Full  arith_type="Signed  (2's comp)"  n_bits=8  bin_pt=2  quantization=Truncate  overflow=Wrap  latency=0  explicit_period=off  period=1  en=off  dbl_ovrd=off  show_param=off  mux_type=off  use_rpm=off  gen_core=off
      settings: xl_area=[0, 0, 0, 0, 0, 0, 0]
  Register : xbsIndex_r3/Register  init=0  reg_only_valid=off  explicit_period=off  period=1  rst=on  en=on  out_en=off  dbl_ovrd=off  show_param=off
      settings: xl_area=[0, 0, 0, 0, 0, 0, 0]
  Slice1 : xbsIndex_r3/Slice  mode=Lower Bit Location + Width  nbits=1  bit1=0  base1=MSB of Input  bit0=4  base0=LSB of Input  boolean_output=on  explicit_period=off  period=1  dbl_ovrd=off
  Slice2 : xbsIndex_r3/Slice  mode=Lower Bit Location + Width  nbits=1  bit1=0  base1=MSB of Input  bit0=0  base0=LSB of Input  boolean_output=on  explicit_period=off  period=1  dbl_ovrd=off
  Slice3 : xbsIndex_r3/Slice  mode=Lower Bit Location + Width  nbits=1  bit1=0  base1=MSB of Input  bit0=3  base0=LSB of Input  boolean_output=on  explicit_period=off  period=1  dbl_ovrd=off
  Slice4 : xbsIndex_r3/Slice  mode=Lower Bit Location + Width  nbits=1  bit1=0  base1=MSB of Input  bit0=2  base0=LSB of Input  boolean_output=on  explicit_period=off  period=1  dbl_ovrd=off
  Slice5 : xbsIndex_r3/Slice  mode=Lower Bit Location + Width  nbits=1  bit1=0  base1=MSB of Input  bit0=1  base0=LSB of Input  boolean_output=on  explicit_period=off  period=1  dbl_ovrd=off
  Slice6 : xbsIndex_r3/Slice  mode=Lower Bit Location + Width  nbits=1  bit1=0  base1=MSB of Input  bit0=0  base0=LSB of Input  boolean_output=on  explicit_period=off  period=1  dbl_ovrd=off
  Slice7 : xbsIndex_r3/Slice  mode=Lower Bit Location + Width  nbits=1  bit1=0  base1=MSB of Input  bit0=5  base0=LSB of Input  boolean_output=on  explicit_period=off  period=1  dbl_ovrd=off
  generate_pulses : Subsystem
  group_period : xps_library/software register  Tag=xps:sw_reg  io_dir=From Processor  arith_type=Unsigned  bitwidth=32  bin_pt=0  sample_period=1  gw_name=b_2x_8a_r309b_dram_tvg2_group_period_user_data_out
  inject_vector : Subsystem  mask{num_vectors=len}
      mask prompts: num_vectors "number of vectors"
      mask init:
      | fmtstr = sprintf('Vector Length: %d', num_vectors);
      | set_param(gcb, 'AttributesFormatString', fmtstr);
      settings: AttributesFormatString=Vector Length: 18432
  inject_vector_location : xps_library/software register  Tag=xps:sw_reg  io_dir=From Processor  arith_type=Unsigned  bitwidth=32  bin_pt=0  sample_period=1  gw_name=b_2x_8a_r309b_dram_tvg2_inject_vector_location_user_data_out
  inject_vector_value : xps_library/software register  Tag=xps:sw_reg  io_dir=From Processor  arith_type=Unsigned  bitwidth=32  bin_pt=0  sample_period=1  gw_name=b_2x_8a_r309b_dram_tvg2_inject_vector_value_user_data_out
  insert_counter : Subsystem  mask{vec_len=len}
      mask prompts: vec_len "Vector Length?"
      mask init:
      | fmtstr = sprintf('Vector Length: %d', vec_len);
      | set_param(gcb, 'AttributesFormatString', fmtstr);
      settings: AttributesFormatString=Vector Length: 18432
  master_reset_sim{1..4} (4 alike) : Constant  Value=0
  master_reset_sim10 : Constant  Value=1000
  master_reset_sim11 : Constant  Value=5
  master_reset_sim5 : Constant
  master_reset_sim7 : Constant  Value=36000000
  master_reset_sim8 : Constant  Value=72
  master_reset_sim9 : Constant  Value=1024
  num_per_group : xps_library/software register  Tag=xps:sw_reg  io_dir=From Processor  arith_type=Unsigned  bitwidth=32  bin_pt=0  sample_period=1  gw_name=b_2x_8a_r309b_dram_tvg2_num_per_group_user_data_out
  num_pulses : xps_library/software register  Tag=xps:sw_reg  io_dir=From Processor  arith_type=Unsigned  bitwidth=32  bin_pt=0  sample_period=1  gw_name=b_2x_8a_r309b_dram_tvg2_num_pulses_user_data_out
  posedge : casper_library/Misc/posedge  Tag=Rising Edge Detector
  rst_vbs : xps_library/software register  Tag=xps:sw_reg  io_dir=From Processor  arith_type=Unsigned  bitwidth=32  bin_pt=0  sample_period=1  gw_name=b_2x_8a_r309b_dram_tvg2_rst_vbs_user_data_out
  valid_bet_sync5 : Subsystem
  valid_bet_sync_sync : Subsystem
  vbs_dram : xps_library/software register  Tag=xps:sw_reg  io_dir=To Processor  arith_type=Unsigned  bitwidth=32  bin_pt=0  sample_period=1  gw_name=b_2x_8a_r309b_dram_tvg2_vbs_dram_user_data_in
  vbs_gen : xps_library/software register  Tag=xps:sw_reg  io_dir=To Processor  arith_type=Unsigned  bitwidth=32  bin_pt=0  sample_period=1  gw_name=b_2x_8a_r309b_dram_tvg2_vbs_gen_user_data_in
  write1 : xps_library/software register  Tag=xps:sw_reg  io_dir=From Processor  arith_type=Unsigned  bitwidth=32  bin_pt=0  sample_period=1  gw_name=b_2x_8a_r309b_dram_tvg2_write1_user_data_out
  write2 : xps_library/software register  Tag=xps:sw_reg  io_dir=From Processor  arith_type=Unsigned  bitwidth=32  bin_pt=0  sample_period=1  gw_name=b_2x_8a_r309b_dram_tvg2_write2_user_data_out
  write3 : xps_library/software register  Tag=xps:sw_reg  io_dir=From Processor  arith_type=Unsigned  bitwidth=32  bin_pt=0  sample_period=1  gw_name=b_2x_8a_r309b_dram_tvg2_write3_user_data_out
  write4 : xps_library/software register  Tag=xps:sw_reg  io_dir=From Processor  arith_type=Unsigned  bitwidth=32  bin_pt=0  sample_period=1  gw_name=b_2x_8a_r309b_dram_tvg2_write4_user_data_out
  new_acc : Outport
  data_out : Outport  Port=2
  valid_out : Outport  Port=3
  wires:
  write1/1 -> Concat/1
  master_reset_sim1/1 -> write1/1
  write2/1 -> Concat/2
  master_reset_sim2/1 -> write2/1
  write3/1 -> Concat/3
  master_reset_sim3/1 -> write3/1
  write4/1 -> Concat/4
  master_reset_sim5/1 -> write4/1
  [new_acc] -> posedge/1
  num_pulses/1 -> generate_pulses/2(num_pulses)
  master_reset_sim7/1 -> num_pulses/1
  num_per_group/1 -> generate_pulses/3(num_per_group)
  master_reset_sim8/1 -> num_per_group/1
  group_period/1 -> generate_pulses/4(group period)
  master_reset_sim9/1 -> group_period/1
  Mux1/1 -> insert_counter/3(valid_in)
  valid_in/1 -> Mux1/2
  inject_vector/1(new_acc_out) -> new_acc/1, valid_bet_sync_sync/1(sync)
  inject_vector/2(data) -> data_out/1
  inject_vector/3(valid_out) -> valid_out/1, valid_bet_sync_sync/3(valid)
  insert_counter/1(new_acc_out) -> inject_vector/1(new_acc_in)
  Mux2/1 -> insert_counter/2(din)
  data_in/1 -> Mux2/2
  new_acc_in/1 -> Mux3/2
  Mux3/1 -> insert_counter/1(new_acc_in)
  Slice5/1 -> [data_sel]
  tvg_sel/1 -> Slice5/1, Slice3/1, Slice1/1, Slice7/1, Slice4/1, Slice6/1
  Slice4/1 -> [valid_sel]
  [valid_sel] -> Mux3/1
  [data_sel] -> Mux2/1
  [valid_sel] -> Mux1/1
  Slice3/1 -> [inj_vector]
  Slice1/1 -> [inj_counter]
  [enable] -> Delay/1
  insert_counter/2(dout) -> inject_vector/2(data_in)
  insert_counter/3(valid_out) -> inject_vector/3(valid_in)
  Concat/1 -> Mux2/3
  generate_pulses/1(valid) -> Register/2, Mux1/3, valid_bet_sync5/3(valid)
  Register/1 -> Mux3/3
  posedge/1 -> Register/1, Register/3, valid_bet_sync5/1(sync)
  [inj_vector] -> inject_vector/6(enable)
  Delay10/1 -> inject_vector/4(vector)
  master_reset_sim11/1 -> inject_vector_location/1
  inject_vector_location/1 -> Delay10/1
  Delay9/1 -> inject_vector/5(value)
  master_reset_sim10/1 -> inject_vector_value/1
  inject_vector_value/1 -> Delay9/1
  [inj_counter] -> insert_counter/4(enable)
  Slice6/1 -> [enable]
  Slice7/1 -> [new_acc]
  valid_bet_sync5/1(max_count) -> vbs_gen/1
  master_reset_sim4/1 -> rst_vbs/1
  Slice2/1 -> valid_bet_sync5/2(rst_max), valid_bet_sync_sync/2(rst_max)
  rst_vbs/1 -> Slice2/1
  valid_bet_sync_sync/1(max_count) -> vbs_dram/1
  Delay/1 -> generate_pulses/1(run)
